simulink model "Lab2_Nhom2_Cau1_3"  (R2025b)
settings: Solver=VariableStepAuto  StartTime=0.0  StopTime=10  RelTol=1e-3

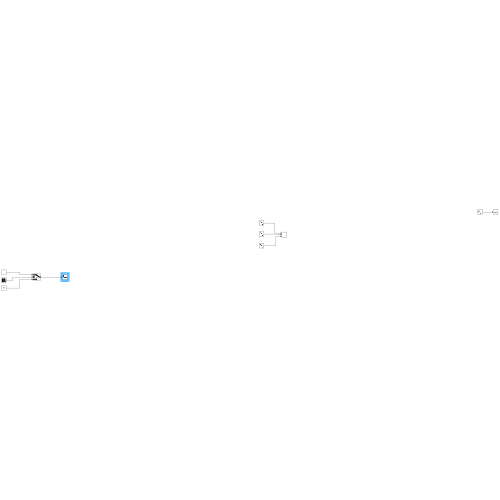
[thumbnail: Simulink's stored preview of the top-level diagram]
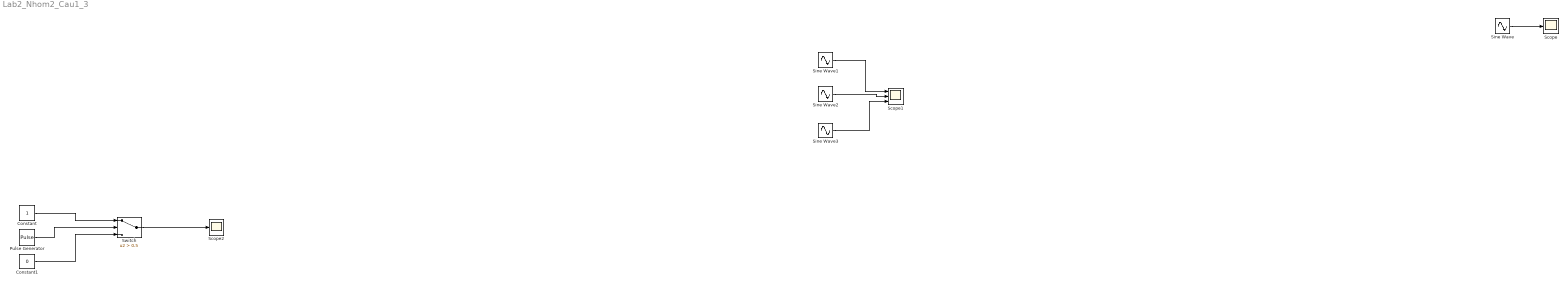
== system Lab2_Nhom2_Cau1_3 ==
  Constant : Constant
  Constant1 : Constant  Value=0
  Pulse Generator : DiscretePulseGenerator  PulseType=Time based  PulseWidth=50
  Scope : Scope
      settings: ActiveDisplayYMinimum=-1.6444734771782197  ActiveDisplayYMaximum=1.7372813408441421
  Scope1 : Scope  NumInputPorts=3
      settings: ActiveDisplayYMinimum=-1.0992785792575039  ActiveDisplayYMaximum=1.233253175473056
  Scope2 : Scope
      settings: ActiveDisplayYMinimum=-0.12499999999999997  ActiveDisplayYMaximum=1.125  DataLoggingVariableName=ScopeData2
  Sine Wave : Sin  Frequency=2*pi*50  Phase=pi/2  SampleTime=0
  Sine Wave1 : Sin  Frequency=50*2*pi  SampleTime=0
  Sine Wave2 : Sin  Frequency=50*2*pi  Phase=pi/2  SampleTime=0
  Sine Wave3 : Sin  Frequency=50*2*pi  Phase=pi  SampleTime=0
  Switch : Switch  Criteria=u2 > Threshold  Threshold=0.5  SaturateOnIntegerOverflow=off  InputSameDT=off
  wires:
  Sine Wave/1 -> Scope/1
  Sine Wave1/1 -> Scope1/1
  Sine Wave2/1 -> Scope1/2
  Sine Wave3/1 -> Scope1/3
  Constant/1 -> Switch/1
  Constant1/1 -> Switch/3
  Pulse Generator/1 -> Switch/2
  Switch/1 -> Scope2/1
